simulink model "ILSGlideslopeSimulink"  (Simulink 10.2)
settings: Solver=VariableStepAuto  StartTime=0.0  StopTime=TF  RelTol=1e-3
values from neighbouring files (symbols this model uses):
  gamma = 3    [ILSGlideslope.m]    (also in Masterscript.m)
  Gamma_ref = 0    [ILSGlideslope.m]    (also in Masterscript.m)
  V_0 = 300    [ILSGlideslope.m]    (also in Masterscript.m)
  w_1 = 0.1    [ILSGlideslope.m]    (also in Masterscript.m)
undefined symbols (not defined in the file or in its folder): magnitude
libraries: pid_lib x2
settings Model: Creator=hooge  LastModifiedBy=hooge
settings DataIOCC: SaveFormat=Dataset  SignalLoggingSaveFormat=Dataset  ReturnWorkspaceOutputs=on
settings OptimizationCC: BlockReduction=off  DefaultParameterBehavior=Inlined  BufferReuse=off  LifeSpan=auto
settings DebuggingCC: UnderspecifiedInitializationDetection=Simplified  MergeDetectMultiDrivingBlocksExec=error  FcnCallInpInsideContextMsg=error  SFUnexpectedBacktrackingDiag=error  SFNoUnconditionalDefaultTransitionDiag=error  SFExecutionAtInitializationDiag=warning  ArithmeticOperatorsInVariantConditions=error
settings HardwareCC: ProdBitPerPointer=64  ProdBitPerSizeT=64  ProdBitPerPtrDiffT=64  ProdLargestAtomicFloat=Float  ProdIntDivRoundTo=Zero  ProdEndianess=LittleEndian  ProdWordSize=64  ProdHWDeviceType=Intel->x86-64 (Windows64)
settings ModelReferenceCC: PropagateSignalLabelsOutOfModel=on
settings SFSimCC: SimUseLocalCustomCode=on  CustomCodeUndefinedFunction=FilterOut
settings RTWCC: RTWUseLocalCustomCode=on
settings CodeAppCC: StateflowObjectComments=off
settings GRTTargetCC: TargetLangStandard=C99 (ISO)  CombineOutputUpdateFcns=on  GRTInterface=off
settings ConfigComp: CovMetricSettings=dwe  CovSaveCumulativeToWorkspaceVar=off  CovSaveSingleToWorkspaceVar=off  CovExternalEMLEnable=on

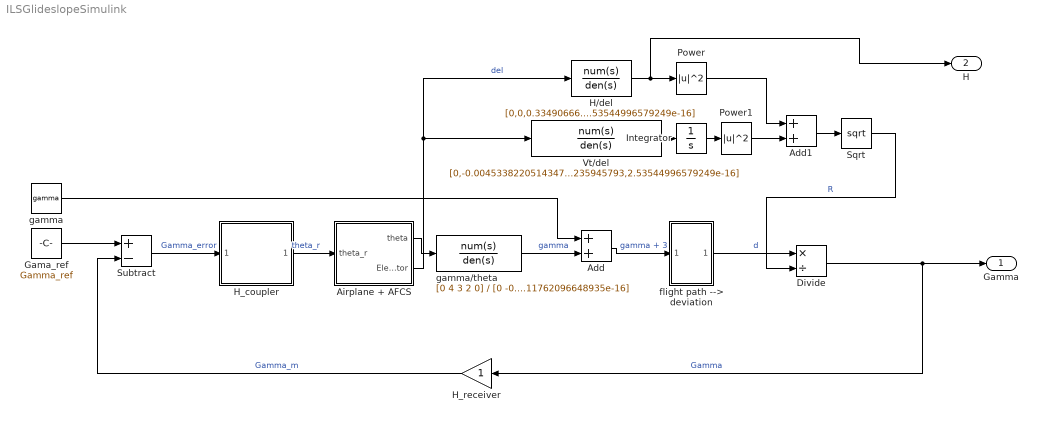
== system ILSGlideslopeSimulink ==
  Add : Sum
  Add1 : Sum
  Airplane + AFCS : Subsystem
  Divide : Product  Inputs=*/
  Gama_ref : Constant  Value=Gamma_ref
  H/del : TransferFcn  Numerator=[0,0,0.334906660037214,-1.16767431772625,-9.42748590867630,0.0841597339239337]  Denominator=[1,1.39070144358098,0.184685132078354,0.00546939746226740,-0.00771920235945793,2.53544996579249e-16]
  H_coupler : Subsystem
  H_receiver : Gain
  Integrator : Integrator
  Power : Math  Operator=magnitude^2  SaturateOnIntegerOverflow=on
  Power1 : Math  Operator=magnitude^2  SaturateOnIntegerOverflow=on
  Sqrt : Sqrt  SaturateOnIntegerOverflow=on
  Subtract : Sum  Inputs=+-
  Vt/del : TransferFcn  Numerator=[0,-0.00453382205143473,0.156520613001318,1.81149513625205,1.01088604649676,0.000380795210759356]  Denominator=[1,1.39070144358098,0.184685132078354,0.00546939746226740,-0.00771920235945793,2.53544996579249e-16]
  flight path --> deviation : Subsystem
  gamma : Constant  Value=gamma
  gamma/theta : TransferFcn  Numerator=[0 4 3 2 0]  Denominator=[0 -0.0570163434913098 -0.0330823046064713 -0.00105185721634336 -4.11762096648935e-16]
  Gamma : Outport
  H : Outport  Port=2
  wires:
  Gama_ref/1 -> Subtract/1
  gamma/1 -> Add/1
  Subtract/1 -> H_coupler/1(gamma_e)  "Gamma_error"
  Airplane + AFCS/1(theta) -> gamma/theta/1
  gamma/theta/1 -> Add/2  "gamma"
  Add/1 -> flight path --> deviation/1(In1)  "gamma + 3"
  flight path --> deviation/1(Out1) -> Divide/1  "d"
  Divide/1 -> Gamma/1, H_receiver/1  "Gamma"
  H_coupler/1(theta_r) -> Airplane + AFCS/1(theta_r)  "theta_r"
  H_receiver/1 -> Subtract/2  "Gamma_m"
  Airplane + AFCS/2(Elevator) -> Vt/del/1, H/del/1  "del"
  Vt/del/1 -> Integrator/1
  Integrator/1 -> Power1/1
  H/del/1 -> H/1, Power/1
  Power/1 -> Add1/1
  Power1/1 -> Add1/2
  Add1/1 -> Sqrt/1
  Sqrt/1 -> Divide/2  "R"

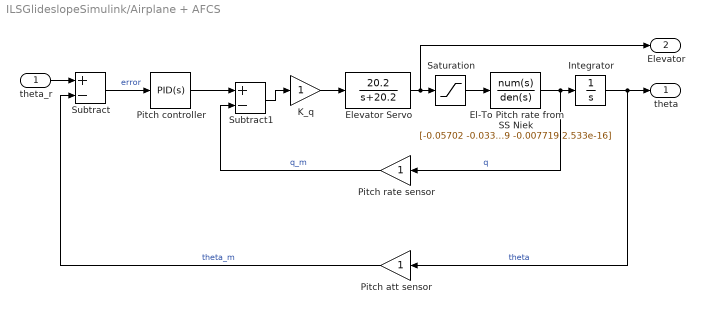
== system ILSGlideslopeSimulink/Airplane + AFCS ==
  theta_r : Inport
  "El-To Pitch rate from SS Niek " : TransferFcn  Numerator=[-0.05702 -0.03308 -0.001052 4.378e-17 0]  Denominator=[1 1.391 0.1847 0.005469 -0.007719 2.533e-16]
  Elevator Servo : TransferFcn  Numerator=[20.2]  Denominator=[1 20.2]
  Integrator : Integrator
  K_q : Gain
  Pitch att sensor : Gain
  Pitch controller : pid_lib/PID Controller  Controller=PID  Form=Parallel  TimeDomain=Continuous-time  UseExternalTs=off  SampleTime=-1  IntegratorMethod=Forward Euler  FilterMethod=Forward Euler  ControllerParametersSource=internal  P=1  I=0  D=1  UseFilter=on  N=100  TunerSelectOption=Transfer Function Based (PID Tuner App)  InitialConditionSource=internal  InitialConditionForIntegrator=0  InitialConditionForFilter=0  DifferentiatorICPrevScaledInput=0  ExternalReset=none  TrackingMode=off  Kt=1  LimitOutput=off  SatLimitsSource=internal  UpperSaturationLimit=inf  LowerSaturationLimit=-inf  LinearizeAsGain=on  AntiWindupMode=none  Kb=1  POutMin=[]  POutMax=[]  IOutMin=[]  IOutMax=[]  DOutMin=[]  DOutMax=[]  NOutMin=[]  NOutMax=[]  SumOutMin=[]  SumOutMax=[]  SaturationOutMin=[]  SaturationOutMax=[]  PParamMin=[]  PParamMax=[]  IParamMin=[]  IParamMax=[]  DParamMin=[]  DParamMax=[]  NParamMin=[]  NParamMax=[]  KbParamMin=[]  KbParamMax=[]  KtParamMin=[]  KtParamMax=[]  KbOutMin=[]  KbOutMax=[]  KtOutMin=[]  KtOutMax=[]  IntegratorOutMin=[]  IntegratorOutMax=[]  FilterOutMin=[]  FilterOutMax=[]  SumI1OutMin=[]  SumI1OutMax=[]  SumI2OutMin=[]  SumI2OutMax=[]  SumI3OutMin=[]  SumI3OutMax=[]  SumI4OutMin=[]  SumI4OutMax=[]  SumDOutMin=[]  SumDOutMax=[]  DifferentiatorOutMin=[]  DifferentiatorOutMax=[]  FilterDiffOutCoefMin=[]  FilterDiffOutCoefMax=[]  ReciprocalOutMin=[]  ReciprocalOutMax=[]  SumDenOutMin=[]  SumDenOutMax=[]  SumNumOutMin=[]  SumNumOutMax=[]  DivideOutMin=[]  DivideOutMax=[]  UdiffTsProdOutMin=[]  UdiffTsProdOutMax=[]  NTsProdOutMin=[]  NTsProdOutMax=[]  UintegralTsProdOutMin=[]  UintegralTsProdOutMax=[]  UngainTsProdOutMin=[]  UngainTsProdOutMax=[]  IntegratorContinuousStateAttributes=''  IntegratorStateMustResolveToSignalObject=off  IntegratorRTWStateStorageClass=Auto  FilterContinuousStateAttributes=''  FilterStateMustResolveToSignalObject=off  FilterRTWStateStorageClass=Auto  ParallelPVariant=InternalParameters  IdealPVariant=Disabled  IVariant=InternalParameters  DVariant=InternalParameters  IntegratorVariant=Continuous  SatVariant=Disabled  AWVariant=Passthrough  PCopyVariant=Disabled  TRVariant=Disabled  FdbkBlocksVariant=Forward  IdealPFdbkVariant=Disabled  SatFdbkVariant=Disabled  DerivativeFilterVariant=ContFilter  NVariant=InternalParameters  NCopyVariant=Disabled  FilterICVariant=InternalICsFilter  IntegratorICVariant=InternalICs  ExternalResetVariant=Disabled  TRSumVariant=Passthrough  SumFdbkVariant=Disabled  SumVariant=Sum_PID  TsampFilterVariant=InternalTs  TsampNgainVariant=Passthrough  TsampIntegralVariant=Passthrough  ExternalSaturationOutDataTypeStr=Inherit: Same as second input
  Pitch rate sensor : Gain
  Saturation : Saturate  UpperLimit=25  LowerLimit=-25
  Subtract : Sum  Inputs=+-
  Subtract1 : Sum  Inputs=+-
  theta : Outport
  Elevator : Outport  Port=2
  wires:
  theta_r/1 -> Subtract/1
  "El-To Pitch rate from SS Niek "/1 -> Pitch rate sensor/1, Integrator/1  "q"
  Integrator/1 -> Pitch att sensor/1, theta/1  "theta"
  Subtract/1 -> Pitch controller/1  "error"
  Pitch controller/1 -> Subtract1/1
  Elevator Servo/1 -> Elevator/1, Saturation/1
  Saturation/1 -> "El-To Pitch rate from SS Niek "/1
  Pitch att sensor/1 -> Subtract/2  "theta_m"
  Subtract1/1 -> K_q/1
  Pitch rate sensor/1 -> Subtract1/2  "q_m"
  K_q/1 -> Elevator Servo/1

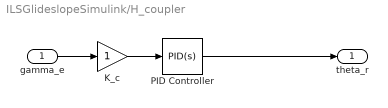
== system ILSGlideslopeSimulink/H_coupler ==
  gamma_e : Inport
  K_c : Gain
  PID Controller : pid_lib/PID Controller  Controller=PID  Form=Parallel  TimeDomain=Continuous-time  UseExternalTs=off  SampleTime=-1  IntegratorMethod=Forward Euler  FilterMethod=Forward Euler  ControllerParametersSource=internal  P=1  I=w_1  D=0  UseFilter=on  N=100  TunerSelectOption=Transfer Function Based (PID Tuner App)  InitialConditionSource=internal  InitialConditionForIntegrator=0  InitialConditionForFilter=0  DifferentiatorICPrevScaledInput=0  ExternalReset=none  TrackingMode=off  Kt=1  LimitOutput=off  SatLimitsSource=internal  UpperSaturationLimit=inf  LowerSaturationLimit=-inf  LinearizeAsGain=on  AntiWindupMode=none  Kb=1  POutMin=[]  POutMax=[]  IOutMin=[]  IOutMax=[]  DOutMin=[]  DOutMax=[]  NOutMin=[]  NOutMax=[]  SumOutMin=[]  SumOutMax=[]  SaturationOutMin=[]  SaturationOutMax=[]  PParamMin=[]  PParamMax=[]  IParamMin=[]  IParamMax=[]  DParamMin=[]  DParamMax=[]  NParamMin=[]  NParamMax=[]  KbParamMin=[]  KbParamMax=[]  KtParamMin=[]  KtParamMax=[]  KbOutMin=[]  KbOutMax=[]  KtOutMin=[]  KtOutMax=[]  IntegratorOutMin=[]  IntegratorOutMax=[]  FilterOutMin=[]  FilterOutMax=[]  SumI1OutMin=[]  SumI1OutMax=[]  SumI2OutMin=[]  SumI2OutMax=[]  SumI3OutMin=[]  SumI3OutMax=[]  SumI4OutMin=[]  SumI4OutMax=[]  SumDOutMin=[]  SumDOutMax=[]  DifferentiatorOutMin=[]  DifferentiatorOutMax=[]  FilterDiffOutCoefMin=[]  FilterDiffOutCoefMax=[]  ReciprocalOutMin=[]  ReciprocalOutMax=[]  SumDenOutMin=[]  SumDenOutMax=[]  SumNumOutMin=[]  SumNumOutMax=[]  DivideOutMin=[]  DivideOutMax=[]  UdiffTsProdOutMin=[]  UdiffTsProdOutMax=[]  NTsProdOutMin=[]  NTsProdOutMax=[]  UintegralTsProdOutMin=[]  UintegralTsProdOutMax=[]  UngainTsProdOutMin=[]  UngainTsProdOutMax=[]  IntegratorContinuousStateAttributes=''  IntegratorStateMustResolveToSignalObject=off  IntegratorRTWStateStorageClass=Auto  FilterContinuousStateAttributes=''  FilterStateMustResolveToSignalObject=off  FilterRTWStateStorageClass=Auto  ParallelPVariant=InternalParameters  IdealPVariant=Disabled  IVariant=InternalParameters  DVariant=InternalParameters  IntegratorVariant=Continuous  SatVariant=Disabled  AWVariant=Passthrough  PCopyVariant=Disabled  TRVariant=Disabled  FdbkBlocksVariant=Forward  IdealPFdbkVariant=Disabled  SatFdbkVariant=Disabled  DerivativeFilterVariant=ContFilter  NVariant=InternalParameters  NCopyVariant=Disabled  FilterICVariant=InternalICsFilter  IntegratorICVariant=InternalICs  ExternalResetVariant=Disabled  TRSumVariant=Passthrough  SumFdbkVariant=Disabled  SumVariant=Sum_PID  TsampFilterVariant=InternalTs  TsampNgainVariant=Passthrough  TsampIntegralVariant=Passthrough  ExternalSaturationOutDataTypeStr=Inherit: Same as second input
  theta_r : Outport
  wires:
  K_c/1 -> PID Controller/1
  PID Controller/1 -> theta_r/1
  gamma_e/1 -> K_c/1

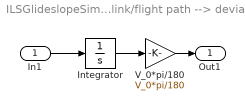
== system ILSGlideslopeSimulink/flight path --> deviation ==
  In1 : Inport
  Integrator : Integrator
  V_0*pi/180 : Gain  Gain=V_0*pi/180
  Out1 : Outport
  wires:
  In1/1 -> Integrator/1
  Integrator/1 -> V_0*pi/180/1
  V_0*pi/180/1 -> Out1/1
